simulink model "mpc_all_constraints_vs_unconstrained"  (R2023a)
settings: Solver=VariableStepAuto  StartTime=0.0  StopTime=0.06  RelTol=1e-3
values from neighbouring files (symbols this model uses):
  B_tilda = [sysdis.B(1) Bw_bar(1,1) Bw_bar(1,2); sysdis.B(2) Bw_bar(2,1) Bw_bar(2,2)]    [motor.m]
  D_tilda = [0 0 0 ; 0 0 0]    [motor.m]
  N = 10    [motor.m]    (also in motor_mpc.m = 3; mpc_unconstrained.m)
  Q_LQ = eye(2)    [motor.m]
  R_LQ = 1    [motor.m]
  sysdis = c2d(sys,Ts)    [motor.m]
  Ts = 0.001    [parameters.m]
  u_max = 12    [constraints.m]
  u_min = 0    [constraints.m]
  uBar = -(A(1,1)*(-A(2,2)*nref/A(2,1)) + A(1,2)*nref)*L    [motor.m]
  w = [1 1]'    [parameters.m]
  x0 = [0.2 70.3]'    [motor.m]
  x_max = [x1_max;x2_max]    [constraints.m]
  x_min = [x1_min;x2_min]    [constraints.m]
  yref = [iref nref]'    [motor.m]
undefined symbols (not defined in the file or in its folder): motor_mpc, motor_mpc_unconstrained, Sd
settings Model: Creator=teora  LastModifiedBy=teora

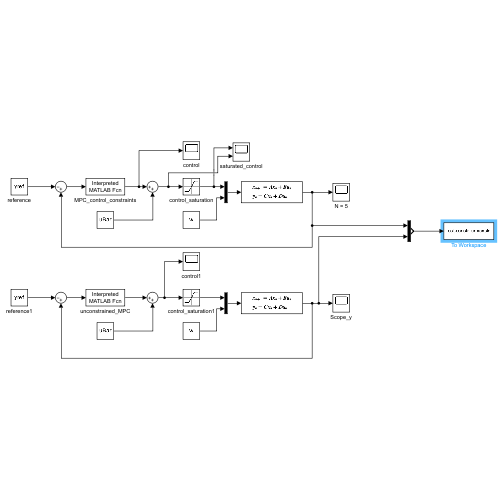
[thumbnail: Simulink's stored preview of the top-level diagram]
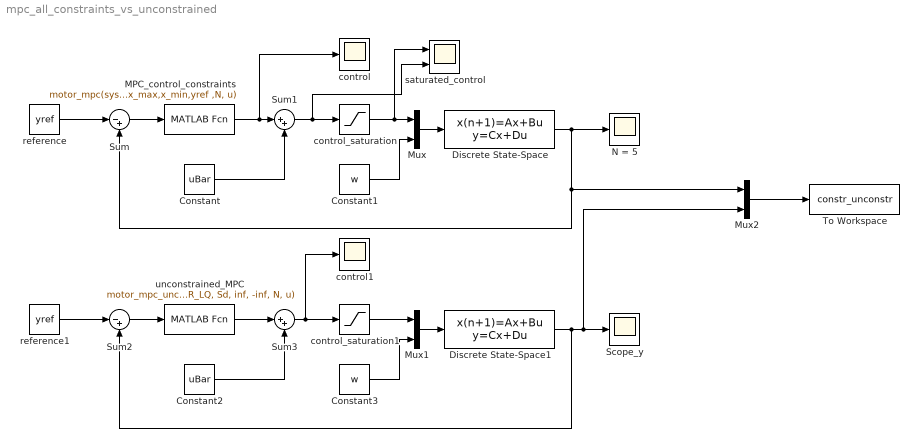
== system mpc_all_constraints_vs_unconstrained ==
  Constant : Constant  Value=uBar
  Constant1 : Constant  Value=w  SampleTime=Ts
  Constant2 : Constant  Value=uBar
  Constant3 : Constant  Value=w
  Discrete State-Space : DiscreteStateSpace  A=sysdis.A  B=B_tilda  C=sysdis.C  D=D_tilda  InitialCondition=x0  SampleTime=Ts
  Discrete State-Space1 : DiscreteStateSpace  A=sysdis.A  B=B_tilda  C=sysdis.C  D=D_tilda  InitialCondition=x0  SampleTime=Ts
  MPC_control_constraints : MATLABFcn  MATLABFcn=motor_mpc(sysdis.A, sysdis.B, Q_LQ, R_LQ, Sd, u_max, u_min, x_max,x_min,yref ,N, u)  OutputDimensions=1
  Mux : Mux  Inputs=2
  Mux1 : Mux  Inputs=2
  Mux2 : Mux  Inputs=2
  N = 5 : Scope
  Scope_y : Scope
  Sum : Sum  Inputs=|-+
  Sum1 : Sum  Inputs=|++
  Sum2 : Sum  Inputs=|-+
  Sum3 : Sum  Inputs=|++
  To Workspace : ToWorkspace  VariableName=constr_unconstr  SaveFormat=Timeseries  SampleTime=-1
  control : Scope
  control1 : Scope
  control_saturation : Saturate  UpperLimit=u_max  LowerLimit=u_min
  control_saturation1 : Saturate  UpperLimit=u_max  LowerLimit=u_min
  reference : Constant  Value=yref
  reference1 : Constant  Value=yref
  saturated_control : Scope  NumInputPorts=2
  unconstrained_MPC : MATLABFcn  MATLABFcn=motor_mpc_unconstrained(sysdis.A, sysdis.B, Q_LQ, R_LQ, Sd, inf, -inf, N, u)  OutputDimensions=1
  wires:
  MPC_control_constraints/1 -> control/1, Sum1/1
  reference/1 -> Sum/1
  control_saturation/1 -> saturated_control/1, Mux/1
  Sum1/1 -> saturated_control/2, control_saturation/1
  Mux/1 -> Discrete State-Space/1
  Sum/1 -> MPC_control_constraints/1
  Constant1/1 -> Mux/2
  Constant/1 -> Sum1/2
  Discrete State-Space/1 -> Mux2/1, Sum/2, N = 5/1
  Mux1/1 -> Discrete State-Space1/1
  Constant2/1 -> Sum3/2
  Constant3/1 -> Mux1/2
  unconstrained_MPC/1 -> Sum3/1
  control_saturation1/1 -> Mux1/1
  reference1/1 -> Sum2/1
  Discrete State-Space1/1 -> Mux2/2, Scope_y/1, Sum2/2
  Sum3/1 -> control1/1, control_saturation1/1
  Sum2/1 -> unconstrained_MPC/1
  Mux2/1 -> To Workspace/1
